simulink model "SpeedControlofBLDCMotorwithPWMusingDriveCycle"  (R2016b)
settings: Solver=ode45  StartTime=0.0  StopTime=13  RelTol=1e-3  EnableMultiTasking=on
undefined symbols (not defined in the file): Ion, Lithium
libraries: powerlib x9, electricdrivelib x2, simulink x2, powerlib_meascontrol x2
settings Model: Creator=Aslam  LastModifiedBy=net
settings DataIOCC: LimitDataPoints=on  SaveFormat=Array
settings OptimizationCC: LifeSpan=inf
settings DebuggingCC: SolverPrmCheckMsg=warning  SFUnexpectedBacktrackingDiag=warning  SFNoUnconditionalDefaultTransitionDiag=warning  SFExecutionAtInitializationDiag=none
settings HardwareCC: ProdBitPerPointer=32  ProdBitPerSizeT=32  ProdBitPerPtrDiffT=32  ProdLargestAtomicFloat=None  ProdIntDivRoundTo=Undefined  ProdEndianess=Unspecified  ProdWordSize=32  ProdHWDeviceType=32-bit Generic
settings ModelReferenceCC: PropagateSignalLabelsOutOfModel=off
settings GRTTargetCC: TargetLangStandard=C89/C90 (ANSI)
settings ConfigComp: CovMetricSettings=dw  CovHtmlReporting=on  CovSaveCumulativeToWorkspaceVar=on  CovSaveSingleToWorkspaceVar=on  CovExternalEMLEnable=off  CovSFcnEnable=off

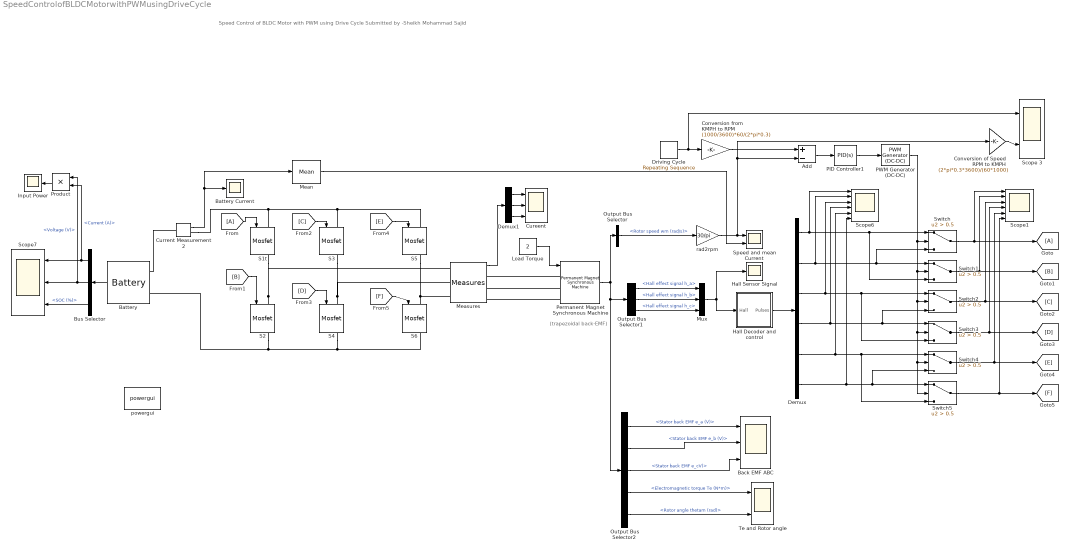
== system SpeedControlofBLDCMotorwithPWMusingDriveCycle ==
  note: Speed Control of BLDC Motor with PWM using Drive Cycle
      | Submitted by -Sheikh Mohammad Sajid
  note: (trapezoidal back-EMF)
  Add : Sum  Inputs=+-
  Back EMF ABC : Scope  NumInputPorts=3
  Battery : electricdrivelib/Extra Sources/Battery  BatType=Lithium-Ion  ShowTempParam=off  ThermalPreset=no  NomV=48  NomQ=6.5  SOC=80  Batt_Tr=30  PresetModel=on  MaxQ=6.5  MinV=36  FullV=55.8714  Dis_rate=2.8261  R=0.073846  Normal_OP=5.8783  expZone="[51.8585     0.319348]"  current=[6.5 13 32.5]  Units=Time  Tci=20  NomT=25  T2=0  MaxQ2=2.208  FullV2=3.45  Normal_OP2=2.8  expZone2="[3.22        0.23]"  Rca=0.6  ti=1000  Dp=0
  Battery Current : Scope
  Bus Selector : BusSelector  OutputSignals=Current (A),Voltage (V),SOC (%)
  "Conversion from KMPH to RPM " : Gain  Gain=(1000/3600)*60/(2*pi*0.3)
  Conversion of Speed RPM to KMPH : Gain  Gain=(2*pi*0.3*3600)/(60*1000)  SaturateOnIntegerOverflow=on  OutDataTypeStr=Inherit: Same as input  ParamDataTypeStr=Inherit: Same as input
  Cureent : Scope  NumInputPorts=3
  Current Measurement2 : powerlib/Measurements/Current Measurement  PhasorSimulation=off  OutputType=Complex  PSBequivalent=0
  Demux : Demux  Outputs=6
  Demux1 : Demux  Outputs=3
  Driving Cycle : simulink/Sources/Repeating Sequence  rep_seq_t=[0 1 2 3 4 5 6 7 8 9 10 11 11.0001 12 13]  rep_seq_y=[0 0 10 10 0 0 20 20 0 0 35 35 25 25 0]
  Hall Decoder and control : Subsystem
  Hall Sensor Signal : Scope
  Input Power : Scope
  Load Torque : Constant  Value=2
  Mean : powerlib_meascontrol/Measurements/Mean  Freq=50  Vinit=0  Ts=0
  Measures : electricdrivelib/AC drives/Brushless DC Motor Drive/Measures
  Mux : Mux  Inputs=3
  Output Bus Selector : BusSelector  OutputSignals=Rotor speed wm (rad/s)
  Output Bus Selector1 : BusSelector  OutputSignals=Hall effect signal h_a,Hall effect signal h_b,Hall effect signal h_c
  Output Bus Selector2 : BusSelector  OutputSignals=Stator back EMF e_a (V),Stator back EMF e_b (V),Stator back EMF e_cV),Electromagnetic torque Te (N*m),Rotor angle thetam (rad)
  PID Controller1 : simulink/Continuous/PID Controller  Controller=PID  TimeDomain=Continuous-time  SampleTime=-1  IntegratorMethod=Forward Euler  FilterMethod=Forward Euler  Form=Parallel  UseFilter=on  ControllerParametersSource=internal  P=1  I=1  D=0  N=100  InitialConditionSource=internal  InitialConditionForIntegrator=0  InitialConditionForFilter=0  ExternalReset=none  LimitOutput=off  UpperSaturationLimit=inf  LowerSaturationLimit=-inf  LinearizeAsGain=on  AntiWindupMode=none  Kb=1  TrackingMode=off  Kt=1  PParamMin=[]  PParamMax=[]  IParamMin=[]  IParamMax=[]  DParamMin=[]  DParamMax=[]  NParamMin=[]  NParamMax=[]  KbParamMin=[]  KbParamMax=[]  KtParamMin=[]  KtParamMax=[]  POutMin=[]  POutMax=[]  IOutMin=[]  IOutMax=[]  DOutMin=[]  DOutMax=[]  NOutMin=[]  NOutMax=[]  KbOutMin=[]  KbOutMax=[]  KtOutMin=[]  KtOutMax=[]  IntegratorOutMin=[]  IntegratorOutMax=[]  FilterOutMin=[]  FilterOutMax=[]  SumOutMin=[]  SumOutMax=[]  SumI1OutMin=[]  SumI1OutMax=[]  SumI2OutMin=[]  SumI2OutMax=[]  SumI3OutMin=[]  SumI3OutMax=[]  SumDOutMin=[]  SumDOutMax=[]  SaturationOutMin=[]  SaturationOutMax=[]  IntegratorContinuousStateAttributes=''  IntegratorStateMustResolveToSignalObject=off  IntegratorRTWStateStorageClass=Auto  FilterContinuousStateAttributes=''  FilterStateMustResolveToSignalObject=off  FilterRTWStateStorageClass=Auto  DifferentiatorICPrevScaledInput=0  DifferentiatorOutMin=[]  DifferentiatorOutMax=[]
  PWM Generator (DC-DC) : powerlib_meascontrol/Pulse & Signal Generators/PWM Generator (DC-DC)  Fsw=5000  Ts=0
  Permanent Magnet Synchronous Machine : powerlib/Machines/Permanent Magnet Synchronous Machine  NbPhases=3  FluxDistribution=Trapezoidal  RotorType=Round  MechanicalLoad=Torque Tm  PresetModel=No  ShowDetailedParameters=on  MeasurementBus=off  Resistance=0.2  Inductance=8.5e-3  dqInductances=[8.5e-3,8.5e-3]  La=0.000835  MachineConstant=Flux linkage established by magnets (V.s)  Flux=0.175  VoltageCst=146.6077  TorqueCst=1.4  Flat=120  Mechanical=[0.12,0.005,4]  PolePairs=4  InitialConditions=[0,0,0,0]  InitialConditions5ph=[0 0 0 0 0 0]  TsPowergui=0  TsBlock=-1  RefAngle=90 degrees behind phase A axis (modified Park)
  Product : Product
  S1t : powerlib/Power Electronics/Mosfet  Ron=0.1  Lon=0  Rd=0.01  Vfd=0  IC=0  Rs=1e5  Cs=inf  Measurements=on
  S{2..6} (5 alike) : powerlib/Power Electronics/Mosfet  Ron=0.1  Lon=0  Rd=0.01  Vfd=0  IC=0  Rs=1e5  Cs=inf  Measurements=on
  Scope 3 : Scope  NumInputPorts=2
  Scope1 : Scope  NumInputPorts=6
  Scope6 : Scope  NumInputPorts=6
  Scope7 : Scope  NumInputPorts=3
  Speed and mean Current : Scope  NumInputPorts=2
  Switch{,1..5} (6 alike) : Switch  Criteria=u2 > Threshold  Threshold=0.5
  Te and Rotor angle : Scope  NumInputPorts=2
  powergui : powerlib/powergui  Priority=1  SimulationMode=Discrete  SolverType=Tustin  SampleTime=5e-6  frequency=60  SPID=off  DisableSnubberDevices=off  DisableRonSwitches=off  DisableVfSwitches=off  SwTol=0  DisplayEquations=off  Interpol=off  ExternalGateDelay=off  methode=off  Ts=0  FunctionMessages=off  echomessages=off  HookPort=off  EnableUseOfTLC=off  x0status=blocks  frequencyindice=0  Pbase=100e6  ErrMax=1e-4  Iterations=50  UnitsV=kV  UnitsW=MW  buscounter=0  RestoreLinks=warning  ResistiveCurrentMeasurement=off  Frange=[0:2:500]  Ylog=off  Xlog=on  ShowGrid=off  save=off  variable=ZData  structure=0  ZoomFFT=off  StartTime=0.0  cycles=1  DisplayStyle=1  fundamental=60  FreqAxis=off  MaxFrequency=1000  frequencyindicesteady=1  RmsSteady=1  display=off
  rad2rpm : Gain  Gain=30/pi  SaturateOnIntegerOverflow=on  OutDataTypeStr=Inherit: Same as input  ParamDataTypeStr=Inherit: Same as input
  wires:
  Permanent Magnet Synchronous Machine/1 -> Output Bus Selector/1, Output Bus Selector2/1, Output Bus Selector1/1
  Load Torque/1 -> Permanent Magnet Synchronous Machine/1
  Output Bus Selector/1 -> rad2rpm/1  "<Rotor speed wm (rad/s)>"
  rad2rpm/1 -> Conversion of Speed RPM to KMPH/1, Add/2, Speed and mean Current/1
  Output Bus Selector1/1 -> Mux/1  "<Hall effect signal h_a>"
  Output Bus Selector1/2 -> Mux/2  "<Hall effect signal h_b>"
  Output Bus Selector1/3 -> Mux/3  "<Hall effect signal h_c>"
  Mux/1 -> Hall Decoder and control/1("Hall "), Hall Sensor Signal/1
  Hall Decoder and control/1(Pulses) -> Demux/1
  Current Measurement2/1 -> Mean/1, Battery Current/1
  [A] -> S1t/1
  [B] -> S2/1
  [C] -> S3/1
  [D] -> S4/1
  [E] -> S5/1
  [F] -> S6/1
  Demux/4 -> Switch2/3, Switch3/1, Scope6/4
  Mean/1 -> Speed and mean Current/2
  Battery/1 -> Bus Selector/1
  Bus Selector/1 -> Scope7/1, Product/2  "<Current (A)>"
  Bus Selector/2 -> Product/1, Scope7/2  "<Voltage (V)>"
  Bus Selector/3 -> Scope7/3  "<SOC (%)>"
  Output Bus Selector2/1 -> Back EMF ABC/1  "<Stator back EMF e_a (V)>"
  Output Bus Selector2/2 -> Back EMF ABC/2  "<Stator back EMF e_b (V)>"
  Output Bus Selector2/3 -> Back EMF ABC/3  "<Stator back EMF e_cV)>"
  Output Bus Selector2/4 -> Te and Rotor angle/1  "<Electromagnetic torque Te (N*m)>"
  Output Bus Selector2/5 -> Te and Rotor angle/2  "<Rotor angle thetam (rad)>"
  Product/1 -> Input Power/1
  Measures/1 -> Demux1/1
  Demux1/1 -> Cureent/1
  Demux1/2 -> Cureent/2
  Demux1/3 -> Cureent/3
  Demux/5 -> Switch5/3, Switch4/1, Scope6/5
  Demux/6 -> Switch4/3, Switch5/1, Scope6/6
  Demux/3 -> Switch3/3, Switch2/1, Scope6/3
  Demux/1 -> Switch1/3, Switch/1, Scope6/1
  Demux/2 -> Switch/3, Switch1/1, Scope6/2
  Switch5/1 -> Scope1/6, [F]
  Switch4/1 -> Scope1/5, [E]
  Switch3/1 -> Scope1/4, [D]
  Switch2/1 -> Scope1/3, [C]
  Switch1/1 -> Scope1/2, [B]
  Switch/1 -> Scope1/1, [A]
  Add/1 -> PID Controller1/1
  "Conversion from KMPH to RPM "/1 -> Add/1
  PID Controller1/1 -> PWM Generator (DC-DC)/1
  PWM Generator (DC-DC)/1 -> Switch5/2, Switch4/2, Switch3/2, Switch2/2, Switch1/2, Switch/2
  Driving Cycle/1 -> Scope 3/1, "Conversion from KMPH to RPM "/1
  Conversion of Speed RPM to KMPH/1 -> Scope 3/2
  connections:
  S2/LConn1 -- S1t/RConn1 -- Measures/LConn1
  S4/LConn1 -- S3/RConn1 -- Measures/LConn2
  S6/LConn1 -- S5/RConn1 -- Measures/LConn3
  Current Measurement2/RConn1 -- S1t/LConn1 -- S3/LConn1 -- S5/LConn1
  S2/RConn1 -- S4/RConn1 -- S6/RConn1 -- Battery/LConn2
  Permanent Magnet Synchronous Machine/LConn2 -- Measures/RConn2
  Permanent Magnet Synchronous Machine/LConn3 -- Measures/RConn3
  Permanent Magnet Synchronous Machine/LConn1 -- Measures/RConn1
  Current Measurement2/LConn1 -- Battery/LConn1

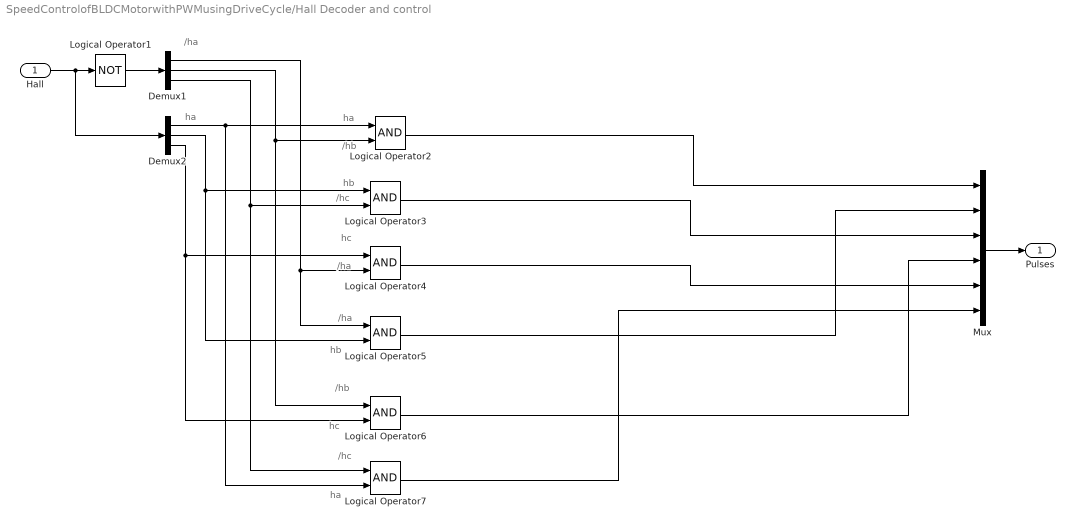
== system SpeedControlofBLDCMotorwithPWMusingDriveCycle/Hall Decoder and control ==
  note: ha
  note: /hc
  note: hc
  note: /hb
  note: hb
  note: /ha
  note: /ha
  note: hc
  note: /hc
  note: hb
  note: /hb
  note: ha
  note: ha
  note: /ha
  "Hall " : Inport
  Demux1 : Demux  Outputs=3
  Demux2 : Demux  Outputs=3
  Logical Operator1 : Logic  Operator=NOT  AllPortsSameDT=off  OutDataTypeStr=boolean
  Logical Operator{2..7} (6 alike) : Logic  AllPortsSameDT=off  OutDataTypeStr=boolean
  Mux : Mux  Inputs=6
  Pulses : Outport
  wires:
  Demux1/3 -> Logical Operator7/1, Logical Operator3/2
  "Hall "/1 -> Demux2/1, Logical Operator1/1
  Demux1/1 -> Logical Operator5/1, Logical Operator4/2
  Demux2/1 -> Logical Operator7/2, Logical Operator2/1
  Demux1/2 -> Logical Operator6/1, Logical Operator2/2
  Demux2/2 -> Logical Operator5/2, Logical Operator3/1
  Logical Operator1/1 -> Demux1/1
  Demux2/3 -> Logical Operator6/2, Logical Operator4/1
  Mux/1 -> Pulses/1
  Logical Operator2/1 -> Mux/1
  Logical Operator3/1 -> Mux/3
  Logical Operator4/1 -> Mux/5
  Logical Operator5/1 -> Mux/2
  Logical Operator6/1 -> Mux/4
  Logical Operator7/1 -> Mux/6
